simulink model "Simu_Design_Model_trim_2014"  (R2014b)
settings: Solver=ode45  StartTime=0.0  StopTime=10000  RelTol=1e-3
InitFcn:
  | load UAV_parameters
  | compute_trim
  | compute_ss_model
  | compute_tf_model
  | addpath('../parameters/')
  | simulation_parameters
  | wind_parameters
  | 
  | save simulink_linear_model  A_lon B_lon A_lat B_lat T_phi_delta_a T_chi_phi T_theta_delta_e T_h_theta T_h_Va T_Va_delta_t T_Va_theta T_v_delta_r
undefined symbols (not defined in the file): drawAircraft, forces_moments, plotmavstatevariables, u_trim, UAV
settings Model: CovHtmlReporting=off  Creator=beard  LastModifiedBy=h1huang
settings DataIOCC: SignalLoggingSaveFormat=ModelDataLogs
settings OptimizationCC: ExpressionDepthLimit=2147483647  InitFltsAndDblsToZero=on
settings DebuggingCC: UnderspecifiedInitializationDetection=Classic  MergeDetectMultiDrivingBlocksExec=none  FcnCallInpInsideContextMsg=EnableAllAsWarning  FrameProcessingCompatibilityMsg=error  StateNameClashWarn=warning
settings GRTTargetCC: CombineOutputUpdateFcns=off  GRTInterface=on

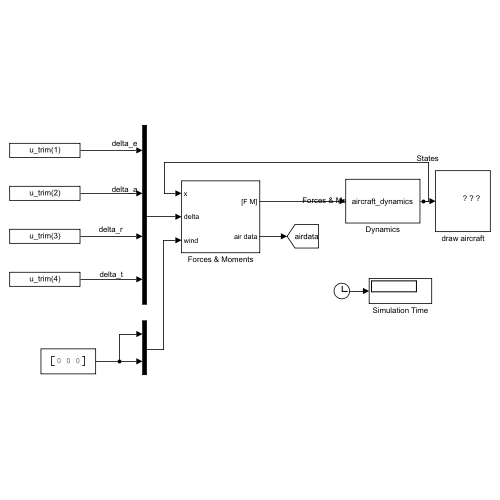
[thumbnail: Simulink's stored preview of the top-level diagram]
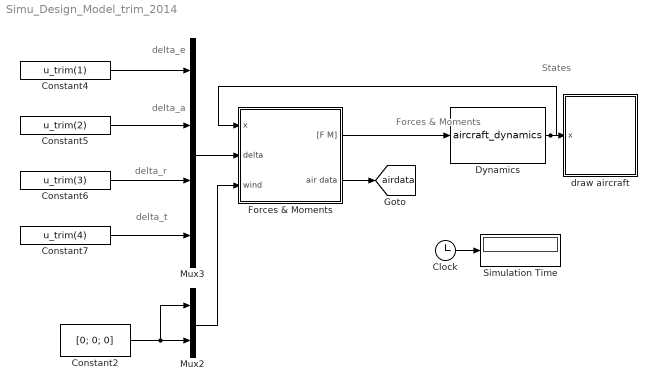
== system Simu_Design_Model_trim_2014 ==
  note: delta_r
  note: delta_t
  note: Forces & Moments
  note: States
  note: delta_e
  note: delta_a
  Clock : Clock
  Constant2 : Constant  Value=[0; 0; 0]
  Constant4 : Constant  Value=u_trim(1)
  Constant5 : Constant  Value=u_trim(2)
  Constant6 : Constant  Value=u_trim(3)
  Constant7 : Constant  Value=u_trim(4)
  Dynamics : S-Function  FunctionName=aircraft_dynamics  Parameters=UAV  SFunctionDeploymentMode=off  EnableBusSupport=off
  Forces & Moments : Subsystem
  Mux2 : Mux  Inputs=2
  Mux3 : Mux
  Simulation Time : Display
  draw aircraft : Subsystem
      mask Display: image(imread('tv.jpg'))
  tag scope: airdata=global
  wires:
  Dynamics/1 -> Forces & Moments/1(x), draw aircraft/1(x)
  Forces & Moments/1("[F M]") -> Dynamics/1
  Clock/1 -> Simulation Time/1
  Forces & Moments/2(air data) -> [airdata]
  Constant2/1 -> Mux2/1, Mux2/2
  Mux3/1 -> Forces & Moments/2(delta)
  Mux2/1 -> Forces & Moments/3(wind)
  Constant4/1 -> Mux3/1
  Constant5/1 -> Mux3/2
  Constant6/1 -> Mux3/3
  Constant7/1 -> Mux3/4

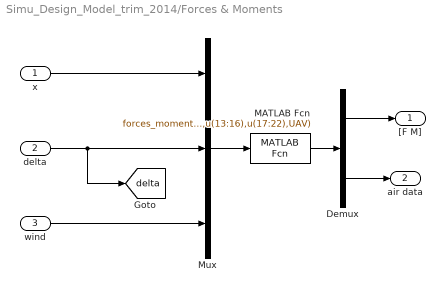
== system Simu_Design_Model_trim_2014/Forces & Moments ==
  x : Inport
  delta : Inport  Port=2
  wind : Inport  Port=3
  Demux : Demux  Outputs=[6;6]
  MATLAB Fcn : MATLABFcn  MATLABFcn=forces_moments(u(1:12),u(13:16),u(17:22),UAV)  OutputDimensions=12
  Mux : Mux  Inputs=3
  "[F M]" : Outport
  air data : Outport  Port=2
  tag scope: delta=global
  wires:
  x/1 -> Mux/1
  delta/1 -> [delta], Mux/2
  wind/1 -> Mux/3
  MATLAB Fcn/1 -> Demux/1
  Demux/1 -> "[F M]"/1
  Mux/1 -> MATLAB Fcn/1
  Demux/2 -> air data/1

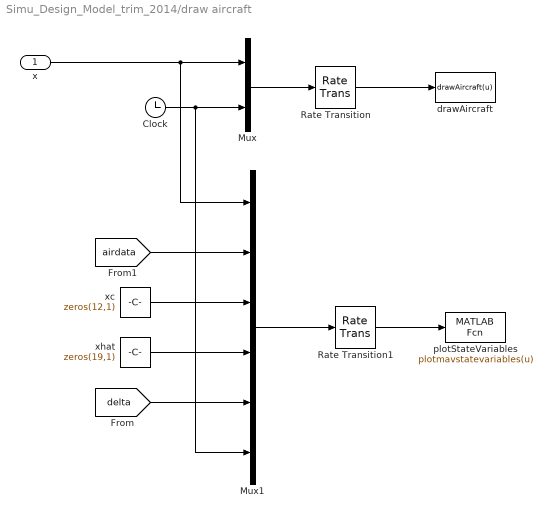
== system Simu_Design_Model_trim_2014/draw aircraft ==
  x : Inport
  Clock : Clock
  Mux : Mux  Inputs=2
  Mux1 : Mux  Inputs=6
  Rate Transition : RateTransition  OutPortSampleTime=SIM.ts_plotting
  Rate Transition1 : RateTransition  OutPortSampleTime=SIM.ts_plotting
  drawAircraft : MATLABFcn  MATLABFcn=drawAircraft(u)  OutputDimensions=0
  plotStateVariables : MATLABFcn  MATLABFcn=plotmavstatevariables(u)  OutputDimensions=0
  xc : Constant  Value=zeros(12,1)
  xhat : Constant  Value=zeros(19,1)
  wires:
  [airdata] -> Mux1/2
  [delta] -> Mux1/5
  xc/1 -> Mux1/3
  xhat/1 -> Mux1/4
  Clock/1 -> Mux1/6, Mux/2
  x/1 -> Mux1/1, Mux/1
  Rate Transition1/1 -> plotStateVariables/1
  Mux1/1 -> Rate Transition1/1
  Mux/1 -> Rate Transition/1
  Rate Transition/1 -> drawAircraft/1
